simulink model "pendulum_model"  (R2022b)
settings: Solver=VariableStepAuto  StartTime=0.0  StopTime=50  RelTol=1e-3
InitFcn:
  | % LRS TU KL %
  | % By Alen Turnwald %
  | % 09.01.2017 %
  | % clc
  | % close
  | 
  | %% g_q
  | % g_q = [1;0];
  | 
  | 
  | % if ~exist('mp','var')||~exist('mc','var')||~exist('L','var')||~exist('g','var')||~exist('d1','var')||~exist('d2','var')
  | % Model Paramter
  |     % warning(['(Some) Model Parameter are not defined!' ,10, '****  Setting the predefined parameter  ****'])
  |     % N = 2;
  |     % mc = 1.5;
  |     % mp = 0.5;
  |     % g = 9.82;
  |     % L = 1;
  | % Damping factors
  |     % d1 = 1e-2;
  |     % d2 = 1e-2;
  | % end
  | 
  | % if ~exist('x_0','var')
  | % Initial state
  |     % warning(['(Initial state "x_0" not defined or wrongly named!' ,10, '****  Setting x_0 = [0.1; 10 deg; 0; 0]  ****'])
  |     % x_0 = zeros(4,1);
  |     % x_0(1) = 0.1;
  |     % x_0(2) = 10*pi/180;
  | % end
  | 
  | % if ~exist('K_lqr','var')||~exist('Kd_lqr','var')
  | %    warning(['(No controller found!' ,10, '****   Applying a predefined controller  ****'])
  | %    K_lqr = [-14.1421  171.8846  -25.2787   54.7535];
  | % end
undefined symbols (not defined in the file or in its folder): A, B, C, disturbance, K_lqr, stall_T, target_angle, x_0
settings Model: Creator=Jake  LastModifiedBy=Jake

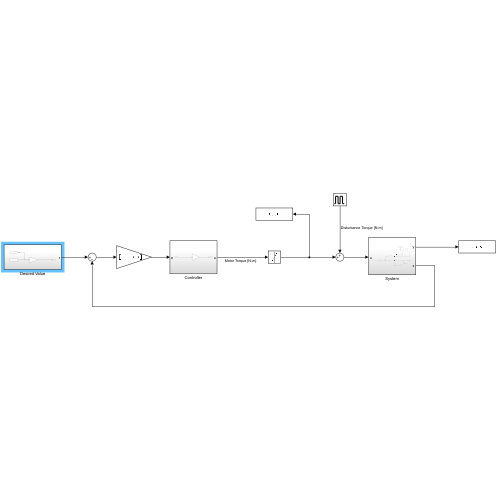
[thumbnail: Simulink's stored preview of the top-level diagram]
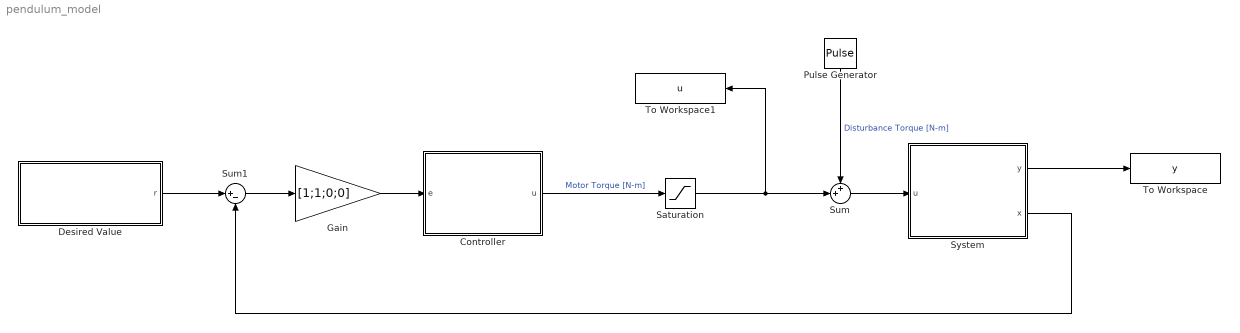
== system pendulum_model ==
  Controller : Subsystem
  Desired Value : Subsystem
  Gain : Gain  Gain=[1;1;0;0]
  Pulse Generator : DiscretePulseGenerator  PulseType=Time based  Amplitude=disturbance  Period=10  PulseWidth=5
  Saturation : Saturate  UpperLimit=stall_T  LowerLimit=-stall_T
  Sum : Sum  Inputs=++|
  Sum1 : Sum  Inputs=|+-
  System : Subsystem
  To Workspace : ToWorkspace  VariableName=y  SampleTime=-1
  To Workspace1 : ToWorkspace  VariableName=u  SampleTime=-1
  wires:
  System/2(x) -> Sum1/2
  System/1(y) -> To Workspace/1
  Controller/1(u) -> Saturation/1  "Motor Torque [N-m]"
  Sum/1 -> System/1(u)
  Saturation/1 -> To Workspace1/1, Sum/2
  Pulse Generator/1 -> Sum/1  "Disturbance Torque [N-m]"
  Desired Value/1(r) -> Sum1/1
  Sum1/1 -> Gain/1
  Gain/1 -> Controller/1(e)

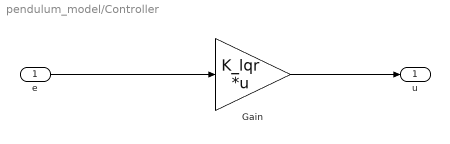
== system pendulum_model/Controller ==
  e : Inport
  Gain : Gain  Gain=K_lqr  Multiplication=Matrix(K*u)
  u : Outport
  wires:
  Gain/1 -> u/1
  e/1 -> Gain/1

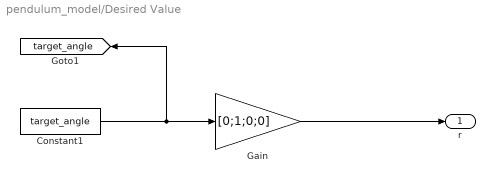
== system pendulum_model/Desired Value ==
  Constant1 : Constant  Value=target_angle
  Gain : Gain  Gain=[0;1;0;0]
  r : Outport
  tag scope: target_angle=global
  wires:
  Constant1/1 -> Gain/1, [target_angle]
  Gain/1 -> r/1

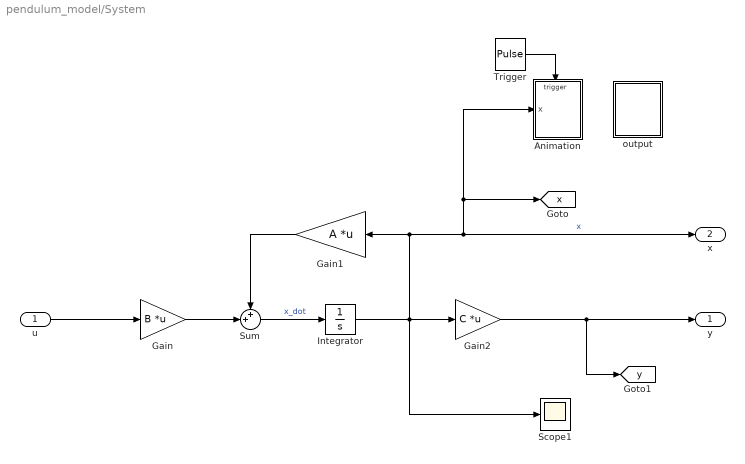
== system pendulum_model/System ==
  u : Inport
  Animation : Subsystem
  Gain : Gain  Gain=B  Multiplication=Matrix(K*u)
  Gain1 : Gain  Gain=A  Multiplication=Matrix(K*u)
  Gain2 : Gain  Gain=C  Multiplication=Matrix(K*u)
  Integrator : Integrator  InitialCondition=x_0
  Scope1 : Scope
  Sum : Sum  Inputs=++|
  Trigger : DiscretePulseGenerator  PulseType=Time based  Period=0.1  PulseWidth=50
  output : Subsystem
  y : Outport
  x : Outport  Port=2
  tag scope: x=global, y=global
  wires:
  u/1 -> Gain/1
  Sum/1 -> Integrator/1  "x_dot"
  Gain2/1 -> y/1, [y]
  Gain1/1 -> Sum/1
  Gain/1 -> Sum/2
  Integrator/1 -> Scope1/1, [x], Animation/1(x), x/1, Gain1/1, Gain2/1  "x"
  Trigger/1 -> Animation/Trigger

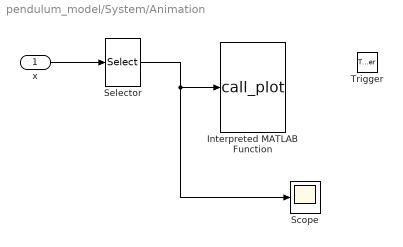
== system pendulum_model/System/Animation ==
  x : Inport
  Trigger : TriggerPort  VariantControl=(inherit)  PortDimensions=1
  Interpreted MATLAB Function : MATLABFcn  MATLABFcn=call_plot  OutputDimensions=0
  Scope : Scope
  Selector : Selector  InputPortWidth=4  IndexOptions=Index vector (dialog)  Indices=[1:2]  OutputSizes=1
  wires:
  x/1 -> Selector/1
  Selector/1 -> Scope/1, Interpreted MATLAB Function/1

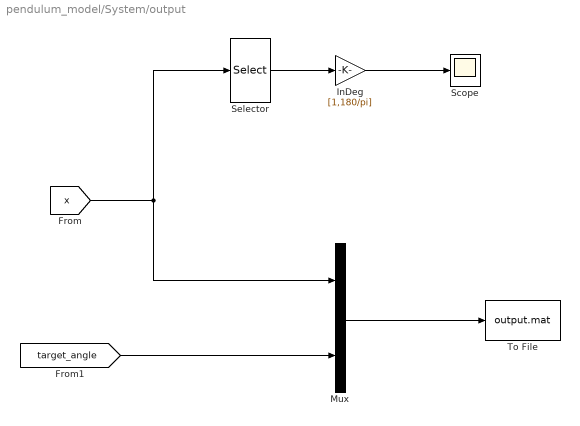
== system pendulum_model/System/output ==
  InDeg : Gain  Gain=[1,180/pi]
  Mux : Mux  Inputs=2
  Scope : Scope
  Selector : Selector  InputPortWidth=4  IndexOptions=Index vector (dialog)  Indices=[1:2]  OutputSizes=1
  To File : ToFile  Filename=output.mat  MatrixName=out  SaveFormat=Timeseries
  wires:
  [x] -> Mux/1, Selector/1
  InDeg/1 -> Scope/1
  Selector/1 -> InDeg/1
  Mux/1 -> To File/1
  [target_angle] -> Mux/2
